simulink model "CAC"  (R2019a)
settings: Solver=VariableStepAuto  StartTime=0.0  StopTime=6  FixedStep=0.001  RelTol=1e-3
values from neighbouring files (symbols this model uses):
  CURRENT_MAX = 3.14    [CAC_ws.mat]    (also in CACu_ws.mat; SimulationParameters.m = 3.14159265359; Simulation_ws.mat = 3.14159265359; TransferFunctions.m = 3.14159265359)
  damping_d = 1.1    [CAC_ws.mat]    (also in CACu_ws.mat = 0.770835010154; abc_ws.mat = 0.770835010154; kalmanSSHumInput.m = 0.9; kalmanStateSpaceModellingHumInput.m = 0.9)
  J_EQ = 0.47    [CAC_ws.mat]    (also in CACu_ws.mat; abc_ws.mat)
  Ki_adm = 1338.03877098    [CAC_ws.mat]    (also in CACu_ws.mat = 1.89921485516; abc_ws.mat = 1.89921485516)
  Kp_adm = 182.625133198    [CAC_ws.mat]    (also in CACu_ws.mat = 0.277331265279; abc_ws.mat = 0.277331265279)
  Ksea = 104    [CAC_ws.mat]    (also in CACu_ws.mat; abc_ws.mat)
  stiffness_d = 0.104    [CAC_ws.mat]    (also in CACu_ws.mat = 14.0803237251; abc_ws.mat = 14.0803237251; kalmanSSHumInput.m = 3.874; kalmanStateSpaceModellingHumInput.m = 3.874)
  Threaded_Ts = 0.001    [CAC_ws.mat]    (also in CACu_ws.mat; SimulationParameters.m; Simulation_ws.mat; abc_ws.mat)
  TORQUE_CONST = 0.0603    [CAC_ws.mat]    (also in CACu_ws.mat; abc_ws.mat)
undefined symbols (not defined in the file or in its folder): DiscIntNeverNeededParam
libraries: simulink x3
settings Model: Creator=Leonardo Felipe  LastModifiedBy=Leonardo Felipe

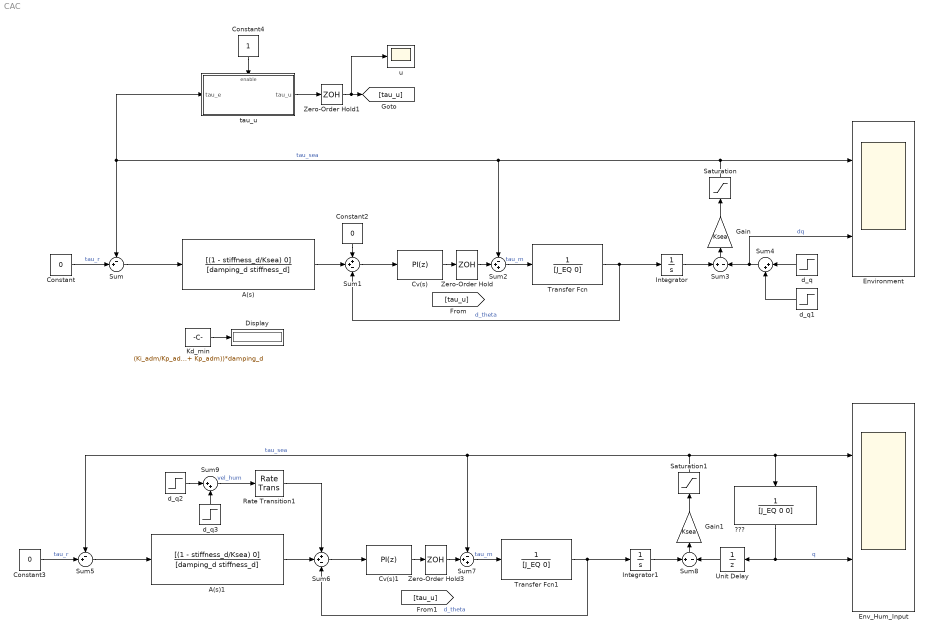
== system CAC ==
  "???" : TransferFcn  Denominator=[J_EQ 0 0]
  A(s) : TransferFcn  Numerator=[(1 - stiffness_d/Ksea) 0]  Denominator=[damping_d stiffness_d]
  A(s)1 : TransferFcn  Numerator=[(1 - stiffness_d/Ksea) 0]  Denominator=[damping_d stiffness_d]
  Constant : Constant  Value=0
  Constant2 : Constant  Value=0
  Constant3 : Constant  Value=0
  Constant4 : Constant  SampleTime=Threaded_Ts
  Cv(s) : simulink/Continuous/PID Controller  Controller=PI  Form=Parallel  TimeDomain=Discrete-time  SampleTime=Threaded_Ts  IntegratorMethod=Forward Euler  FilterMethod=Forward Euler  ControllerParametersSource=internal  P=Kp_adm  I=Ki_adm  D=0  UseFilter=on  N=100  TunerSelectOption=Transfer Function Based (PID Tuner App)  InitialConditionSource=internal  InitialConditionForIntegrator=0  InitialConditionForFilter=0  DifferentiatorICPrevScaledInput=0  ExternalReset=none  TrackingMode=off  Kt=1  LimitOutput=off  UpperSaturationLimit=inf  LowerSaturationLimit=-inf  LinearizeAsGain=on  AntiWindupMode=none  Kb=1  POutMin=[]  POutMax=[]  IOutMin=[]  IOutMax=[]  DOutMin=[]  DOutMax=[]  NOutMin=[]  NOutMax=[]  SumOutMin=[]  SumOutMax=[]  SaturationOutMin=[]  SaturationOutMax=[]  PParamMin=[]  PParamMax=[]  IParamMin=[]  IParamMax=[]  DParamMin=[]  DParamMax=[]  NParamMin=[]  NParamMax=[]  KbParamMin=[]  KbParamMax=[]  KtParamMin=[]  KtParamMax=[]  KbOutMin=[]  KbOutMax=[]  KtOutMin=[]  KtOutMax=[]  IntegratorOutMin=[]  IntegratorOutMax=[]  FilterOutMin=[]  FilterOutMax=[]  SumI1OutMin=[]  SumI1OutMax=[]  SumI2OutMin=[]  SumI2OutMax=[]  SumI3OutMin=[]  SumI3OutMax=[]  SumI4OutMin=[]  SumI4OutMax=[]  SumDOutMin=[]  SumDOutMax=[]  DifferentiatorOutMin=[]  DifferentiatorOutMax=[]  FilterDiffOutCoefMin=[]  FilterDiffOutCoefMax=[]  ReciprocalOutMin=[]  ReciprocalOutMax=[]  SumDenOutMin=[]  SumDenOutMax=[]  SumNumOutMin=[]  SumNumOutMax=[]  DivideOutMin=[]  DivideOutMax=[]  IntegratorContinuousStateAttributes=''  IntegratorStateMustResolveToSignalObject=off  IntegratorRTWStateStorageClass=Auto  FilterContinuousStateAttributes=''  FilterStateMustResolveToSignalObject=off  FilterRTWStateStorageClass=Auto  ParallelPVariant=InternalParameters  IdealPVariant=Disabled  IVariant=InternalParameters  DVariant=Disabled  IntegratorVariant=Discrete  SatVariant=Disabled  AWVariant=Passthrough  PCopyVariant=Disabled  TRVariant=Disabled  FdbkBlocksVariant=Forward  IdealPFdbkVariant=Disabled  SatFdbkVariant=Disabled  DerivativeFilterVariant=Disabled  NVariant=Disabled  NCopyVariant=Disabled_SignalSpec  FilterICVariant=Disabled  IntegratorICVariant=InternalICs  ExternalResetVariant=Disabled  TRSumVariant=Passthrough  SumFdbkVariant=Disabled  SumVariant=Sum_PI
  Cv(s)1 : simulink/Continuous/PID Controller  Controller=PI  Form=Parallel  TimeDomain=Discrete-time  SampleTime=Threaded_Ts  IntegratorMethod=Forward Euler  FilterMethod=Forward Euler  ControllerParametersSource=internal  P=Kp_adm  I=Ki_adm  D=0  UseFilter=on  N=100  TunerSelectOption=Transfer Function Based (PID Tuner App)  InitialConditionSource=internal  InitialConditionForIntegrator=0  InitialConditionForFilter=0  DifferentiatorICPrevScaledInput=0  ExternalReset=none  TrackingMode=off  Kt=1  LimitOutput=off  UpperSaturationLimit=inf  LowerSaturationLimit=-inf  LinearizeAsGain=on  AntiWindupMode=none  Kb=1  POutMin=[]  POutMax=[]  IOutMin=[]  IOutMax=[]  DOutMin=[]  DOutMax=[]  NOutMin=[]  NOutMax=[]  SumOutMin=[]  SumOutMax=[]  SaturationOutMin=[]  SaturationOutMax=[]  PParamMin=[]  PParamMax=[]  IParamMin=[]  IParamMax=[]  DParamMin=[]  DParamMax=[]  NParamMin=[]  NParamMax=[]  KbParamMin=[]  KbParamMax=[]  KtParamMin=[]  KtParamMax=[]  KbOutMin=[]  KbOutMax=[]  KtOutMin=[]  KtOutMax=[]  IntegratorOutMin=[]  IntegratorOutMax=[]  FilterOutMin=[]  FilterOutMax=[]  SumI1OutMin=[]  SumI1OutMax=[]  SumI2OutMin=[]  SumI2OutMax=[]  SumI3OutMin=[]  SumI3OutMax=[]  SumI4OutMin=[]  SumI4OutMax=[]  SumDOutMin=[]  SumDOutMax=[]  DifferentiatorOutMin=[]  DifferentiatorOutMax=[]  FilterDiffOutCoefMin=[]  FilterDiffOutCoefMax=[]  ReciprocalOutMin=[]  ReciprocalOutMax=[]  SumDenOutMin=[]  SumDenOutMax=[]  SumNumOutMin=[]  SumNumOutMax=[]  DivideOutMin=[]  DivideOutMax=[]  IntegratorContinuousStateAttributes=''  IntegratorStateMustResolveToSignalObject=off  IntegratorRTWStateStorageClass=Auto  FilterContinuousStateAttributes=''  FilterStateMustResolveToSignalObject=off  FilterRTWStateStorageClass=Auto  ParallelPVariant=InternalParameters  IdealPVariant=Disabled  IVariant=InternalParameters  DVariant=Disabled  IntegratorVariant=Discrete  SatVariant=Disabled  AWVariant=Passthrough  PCopyVariant=Disabled  TRVariant=Disabled  FdbkBlocksVariant=Forward  IdealPFdbkVariant=Disabled  SatFdbkVariant=Disabled  DerivativeFilterVariant=Disabled  NVariant=Disabled  NCopyVariant=Disabled_SignalSpec  FilterICVariant=Disabled  IntegratorICVariant=InternalICs  ExternalResetVariant=Disabled  TRSumVariant=Passthrough  SumFdbkVariant=Disabled  SumVariant=Sum_PI
  Display : Display
      settings: Decimation=5
  Env_Hum_Input : Scope  NumInputPorts=2
  Environment : Scope  NumInputPorts=2
  Gain : Gain  Gain=Ksea
  Gain1 : Gain  Gain=Ksea
  Integrator : Integrator
  Integrator1 : Integrator
  Kd_min : Constant  Value=(Ki_adm/Kp_adm - 1/J_EQ*(damping_d/(1 - stiffness_d/Ksea) + Kp_adm))*damping_d  SampleTime=0.001
  Rate Transition1 : RateTransition  OutPortSampleTime=Threaded_Ts
  Saturation : Saturate  UpperLimit=250  LowerLimit=-250
  Saturation1 : Saturate  UpperLimit=250  LowerLimit=-250
  Sum : Sum  Inputs=-+|
  Sum1 : Sum  Inputs=++-
  Sum2 : Sum  Inputs=-++
  Sum3 : Sum  Inputs=+-
  Sum4 : Sum  Inputs=|++
  Sum5 : Sum  Inputs=-+|
  Sum6 : Sum  Inputs=++-
  Sum7 : Sum  Inputs=-++
  Sum8 : Sum  Inputs=+-
  Sum9 : Sum  Inputs=|++
  Transfer Fcn : TransferFcn  Denominator=[J_EQ 0]
  Transfer Fcn1 : TransferFcn  Denominator=[J_EQ 0]
  Unit Delay : UnitDelay  SampleTime=-1  HasFrameUpgradeWarning=on
  Zero-Order Hold : ZeroOrderHold  SampleTime=Threaded_Ts
  Zero-Order Hold1 : ZeroOrderHold  SampleTime=Threaded_Ts
  Zero-Order Hold3 : ZeroOrderHold  SampleTime=Threaded_Ts
  d_q : Step  SampleTime=0
  d_q1 : Step  Time=1.4  After=-1  SampleTime=0
  d_q2 : Step  SampleTime=0.008
  d_q3 : Step  Time=1.4  After=-1  SampleTime=0.008
  tau_u : Subsystem
  u : Scope
  wires:
  Sum/1 -> A(s)/1
  Constant/1 -> Sum/2  "tau_r"
  A(s)/1 -> Sum1/2
  Sum1/1 -> Cv(s)/1
  Cv(s)/1 -> Zero-Order Hold/1
  Zero-Order Hold/1 -> Sum2/2
  Sum2/1 -> Transfer Fcn/1  "tau_m"
  Transfer Fcn/1 -> Sum1/3, Integrator/1  "d_theta"
  Sum3/1 -> Gain/1
  Gain/1 -> Saturation/1
  Zero-Order Hold1/1 -> u/1, [tau_u]
  Constant2/1 -> Sum1/1
  tau_u/1(tau_u) -> Zero-Order Hold1/1
  Constant4/1 -> tau_u/Enable
  d_q/1 -> Sum4/1
  d_q1/1 -> Sum4/2
  Saturation/1 -> Environment/1, Sum2/1, Sum/1, tau_u/1(tau_e)  "tau_sea"
  Kd_min/1 -> Display/1
  Sum4/1 -> Environment/2, Sum3/2  "dq"
  Integrator/1 -> Sum3/1
  Integrator1/1 -> Sum8/1
  Saturation1/1 -> Sum5/1, Sum7/1, Env_Hum_Input/1, "???"/1  "tau_sea"
  d_q3/1 -> Sum9/2
  d_q2/1 -> Sum9/1
  Rate Transition1/1 -> Sum6/1
  Gain1/1 -> Saturation1/1
  Sum8/1 -> Gain1/1
  Transfer Fcn1/1 -> Integrator1/1, Sum6/3  "d_theta"
  Sum7/1 -> Transfer Fcn1/1  "tau_m"
  Zero-Order Hold3/1 -> Sum7/2
  Cv(s)1/1 -> Zero-Order Hold3/1
  Sum6/1 -> Cv(s)1/1
  Sum9/1 -> Rate Transition1/1  "vel_hum"
  A(s)1/1 -> Sum6/2
  Constant3/1 -> Sum5/2  "tau_r"
  Sum5/1 -> A(s)1/1
  "???"/1 -> Env_Hum_Input/2, Unit Delay/1  "q"
  Unit Delay/1 -> Sum8/2

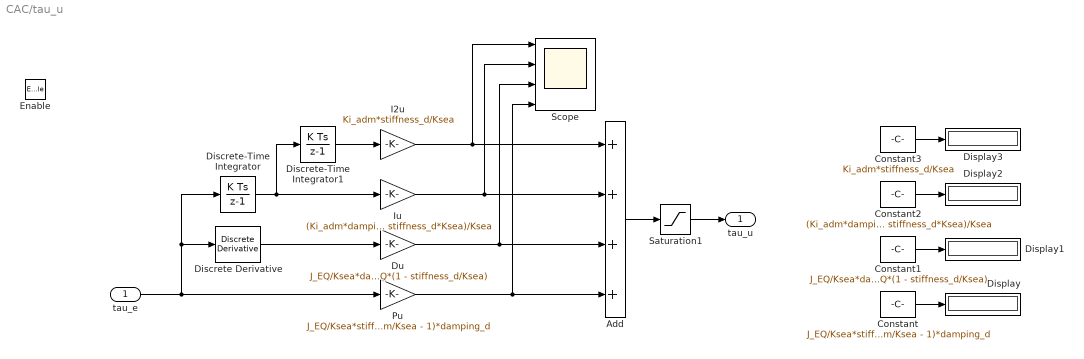
== system CAC/tau_u ==
  tau_e : Inport  SampleTime=0.001
  Enable : EnablePort
  Add : Sum  Inputs=++++
  Constant : Constant  Value=J_EQ/Ksea*stiffness_d + (Kp_adm/Ksea - 1)*damping_d  SampleTime=0.001
  Constant1 : Constant  Value=J_EQ/Ksea*damping_d - J_EQ*(1 - stiffness_d/Ksea)  SampleTime=0.001
  Constant2 : Constant  Value=(Ki_adm*damping_d + Kp_adm*stiffness_d - stiffness_d*Ksea)/Ksea  SampleTime=0.001
  Constant3 : Constant  Value=Ki_adm*stiffness_d/Ksea  SampleTime=0.001
  Discrete Derivative : simulink/Discrete/Discrete Derivative  gainval=1.0  ICPrevScaledInput=0.0  OutMin=[]  OutMax=[]  OutDataType=fixdt(1, 16)  OutScaling=2^-10  DoSatur=off
  Discrete-Time Integrator : DiscreteIntegrator  SampleTime=0.001  ICPrevOutput=DiscIntNeverNeededParam  ICPrevScaledInput=DiscIntNeverNeededParam
  Discrete-Time Integrator1 : DiscreteIntegrator  SampleTime=0.001  ICPrevOutput=DiscIntNeverNeededParam  ICPrevScaledInput=DiscIntNeverNeededParam
  Display{,1..3} (4 alike) : Display
      settings: Decimation=5
  Du : Gain  Gain=J_EQ/Ksea*damping_d - J_EQ*(1 - stiffness_d/Ksea)
  I2u : Gain  Gain=Ki_adm*stiffness_d/Ksea
  Iu : Gain  Gain=(Ki_adm*damping_d + Kp_adm*stiffness_d - stiffness_d*Ksea)/Ksea
  Pu : Gain  Gain=J_EQ/Ksea*stiffness_d + (Kp_adm/Ksea - 1)*damping_d
  Saturation1 : Saturate  UpperLimit=TORQUE_CONST*CURRENT_MAX  LowerLimit=-TORQUE_CONST*CURRENT_MAX
  Scope : Scope  NumInputPorts=4
  tau_u : Outport  SampleTime=0.001
  wires:
  Add/1 -> Saturation1/1
  Du/1 -> Scope/3, Add/3
  Discrete Derivative/1 -> Du/1
  Iu/1 -> Scope/2, Add/2
  Pu/1 -> Scope/4, Add/4
  Discrete-Time Integrator/1 -> Discrete-Time Integrator1/1, Iu/1
  I2u/1 -> Scope/1, Add/1
  Discrete-Time Integrator1/1 -> I2u/1
  tau_e/1 -> Pu/1, Discrete-Time Integrator/1, Discrete Derivative/1
  Saturation1/1 -> tau_u/1
  Constant/1 -> Display/1
  Constant1/1 -> Display1/1
  Constant2/1 -> Display2/1
  Constant3/1 -> Display3/1
